simulink model "UAM_Flight_control"  (R2024b)
settings: Solver=FixedStepAuto  StartTime=0.0  StopTime=inf  RelTol=1e-3  EnableMultiTasking=on
undefined symbols (not defined in the file): CityMission, control, controlParams, ControlSampleTime, Cruise_a, DiscIntNeverNeededParam, Earth, FixedWingMission, flightState, FSState, FWControlParams, FWTrimSpeed, HoverMission, params, position, R_WAYPOINTTRANSITION, TransitionMission, uavParam, Vt, w_trim, WGS84, zGround
libraries: slpidlib x56, simulink x32, uavalgslib x7, robotcorelib x2, simulink_extras x2, mspfiltlib x1, aerolibtransform2 x1
(part 5 of 13)

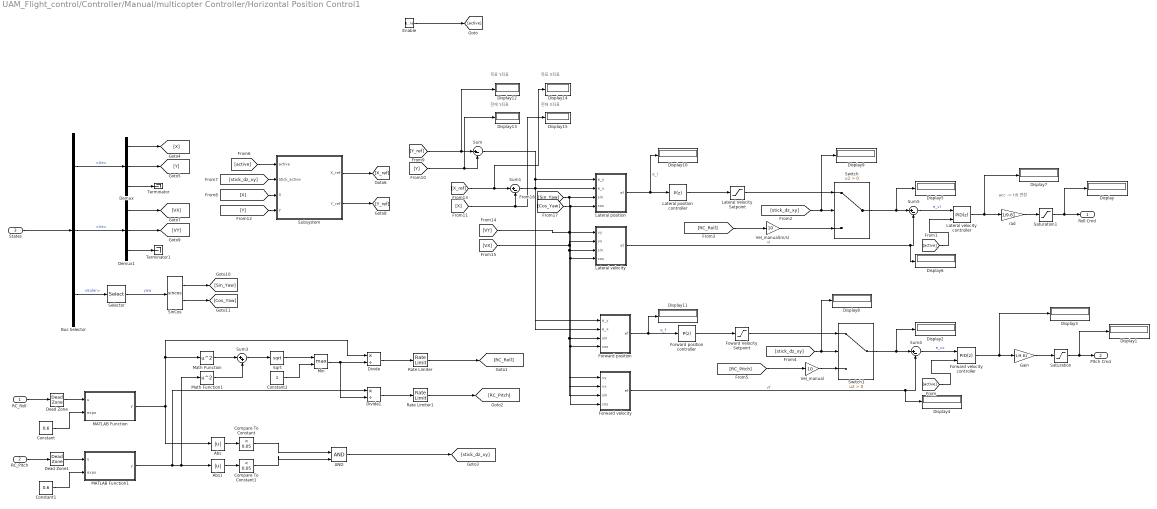
== system UAM_Flight_control/Controller/Manual/multicopter Controller/Horizontal Position Control1 ==
  note: 현재 X좌표
  note: 현재 Y좌표
  note: acc -> tilt 변환
  note: 목표 X좌표
  note: 목표 Y좌표
  RC_Roll : Inport
  RC_Pitch : Inport  Port=2
  States : Inport  Port=3
  Enable : EnablePort  StatesWhenEnabling=reset  ShowOutputPort=on
  AND : Logic  IconShape=distinctive  AllPortsSameDT=off  OutDataTypeStr=boolean
  Abs : Abs  SaturateOnIntegerOverflow=off
  Abs1 : Abs  SaturateOnIntegerOverflow=off
  Bus Selector : BusSelector  OutputSignals=Xe,Ve,Euler
  Compare To Constant : simulink/Logic and Bit Operations/Compare To Constant  relop=<  const=0.05  OutDataTypeStr=boolean
  Compare To Constant1 : simulink/Logic and Bit Operations/Compare To Constant  relop=<  const=0.05  OutDataTypeStr=boolean
  Constant : Constant  Value=0.6
  Constant1 : Constant  Value=0.6
  Constant2 : Constant
  Dead Zone : DeadZone  LowerValue=-0.1  UpperValue=0.1
  Dead Zone1 : DeadZone  LowerValue=-0.1  UpperValue=0.1
  Demux : Demux  Outputs=3
  Demux1 : Demux  Outputs=3
  Display{,1..15} (16 alike) : Display
  Divide : Product  Inputs=*/
  Divide1 : Product  Inputs=*/
  Forward position : Subsystem
  Forward position controller : slpidlib/PID Controller  Controller=P  Form=Parallel  TimeDomain=Discrete-time  UseExternalTs=off  SampleTime=-1  IntegratorMethod=Forward Euler  FilterMethod=Forward Euler  ControllerParametersSource=internal  P=controlParams.P_X  I=controlParams.I_X  UseKiTs=off  D=controlParams.D_X  UseExternalDerivativeSource=off  N=controlParams.N_X  UseFilter=on  TunerSelectOption=Transfer Function Based (PID Tuner App)  InitialConditionSource=internal  InitialConditionForIntegrator=0  InitialConditionForFilter=0  DifferentiatorICPrevScaledInput=0  ExternalReset=none  TrackingMode=off  Kt=1  LimitOutput=off  SatLimitsSource=internal  UpperSaturationLimit=inf  LowerSaturationLimit=-inf  LinearizeAsGain=on  AntiWindupMode=none  Kb=1  LimitIntegrator=off  UpperIntegratorSaturationLimit=inf  LowerIntegratorSaturationLimit=-inf  POutMin=[]  POutMax=[]  IOutMin=[]  IOutMax=[]  DOutMin=[]  DOutMax=[]  NOutMin=[]  NOutMax=[]  SumOutMin=[]  SumOutMax=[]  SaturationOutMin=[]  SaturationOutMax=[]  PParamMin=[]  PParamMax=[]  IParamMin=[]  IParamMax=[]  DParamMin=[]  DParamMax=[]  NParamMin=[]  NParamMax=[]  KbParamMin=[]  KbParamMax=[]  KtParamMin=[]  KtParamMax=[]  KbOutMin=[]  KbOutMax=[]  KtOutMin=[]  KtOutMax=[]  IntegratorOutMin=[]  IntegratorOutMax=[]  FilterOutMin=[]  FilterOutMax=[]  SumI1OutMin=[]  SumI1OutMax=[]  SumI2OutMin=[]  SumI2OutMax=[]  SumI3OutMin=[]  SumI3OutMax=[]  SumI4OutMin=[]  SumI4OutMax=[]  SumDOutMin=[]  SumDOutMax=[]  DifferentiatorOutMin=[]  DifferentiatorOutMax=[]  FilterDiffOutCoefMin=[]  FilterDiffOutCoefMax=[]  ReciprocalOutMin=[]  ReciprocalOutMax=[]  SumDenOutMin=[]  SumDenOutMax=[]  SumNumOutMin=[]  SumNumOutMax=[]  DivideOutMin=[]  DivideOutMax=[]  UdiffTsProdOutMin=[]  UdiffTsProdOutMax=[]  NTsProdOutMin=[]  NTsProdOutMax=[]  UintegralTsProdOutMin=[]  UintegralTsProdOutMax=[]  UngainTsProdOutMin=[]  UngainTsProdOutMax=[]  ClampingZeroOutDataTypeStr=Inherit: Inherit via back propagation  ClampingZeroOutMin=[]  ClampingZeroOutMax=[]  FilterDenConstantOutDataTypeStr=Inherit: Inherit via back propagation  FilterDenConstantOutMin=[]  FilterDenConstantOutMax=[]  PCopyOutDataTypeStr=Inherit: Inherit via back propagation  PCopyOutMin=[]  PCopyOutMax=[]  NCopyOutDataTypeStr=Inherit: Inherit via back propagation  NCopyOutMin=[]  NCopyOutMax=[]  IntegratorContinuousStateAttributes=''  IntegratorStateMustResolveToSignalObject=off  IntegratorRTWStateStorageClass=Auto  FilterContinuousStateAttributes=''  FilterStateMustResolveToSignalObject=off  FilterRTWStateStorageClass=Auto  ParallelPVariant=InternalParameters  IdealPVariant=Disabled  IVariant=Disabled  DVariant=Disabled  IntegratorVariant=Disabled  SatVariant=Disabled  AWVariant=Disabled  PCopyVariant=Disabled  TRVariant=Disabled  FdbkBlocksVariant=Forward  IdealPFdbkVariant=Disabled  SatFdbkVariant=Disabled  DerivativeFilterVariant=Disabled  NVariant=Disabled  NCopyVariant=Disabled_SignalSpec  FilterICVariant=Disabled  IntegratorICVariant=Disabled  ExternalResetVariant=Disabled  TRSumVariant=Passthrough  SumFdbkVariant=Disabled  SumVariant=Passthrough_P  TsampFilterVariant=InternalTs  TsampNgainVariant=Passthrough  TsampIntegralVariant=Disabled_SignalSpec  ExternalSaturationOutDataTypeStr=Inherit: Same as second input  DerivativeSourceVariant=Disabled  PreIntVariant=InternalPreInt
  Forward velocity : Subsystem
  Forward velocity controller : slpidlib/PID Controller  Controller=PID  Form=Parallel  TimeDomain=Discrete-time  UseExternalTs=off  SampleTime=-1  IntegratorMethod=Forward Euler  FilterMethod=Forward Euler  ControllerParametersSource=internal  P=controlParams.P_VX  I=controlParams.I_VX  UseKiTs=off  D=controlParams.D_VX  UseExternalDerivativeSource=off  N=controlParams.N_VX  UseFilter=on  TunerSelectOption=Transfer Function Based (PID Tuner App)  InitialConditionSource=internal  InitialConditionForIntegrator=0  InitialConditionForFilter=0  DifferentiatorICPrevScaledInput=0  ExternalReset=rising  TrackingMode=off  Kt=1  LimitOutput=on  SatLimitsSource=internal  UpperSaturationLimit=5  LowerSaturationLimit=-5  LinearizeAsGain=on  AntiWindupMode=clamping  Kb=1  LimitIntegrator=on  UpperIntegratorSaturationLimit=2  LowerIntegratorSaturationLimit=-2  POutMin=[]  POutMax=[]  IOutMin=[]  IOutMax=[]  DOutMin=[]  DOutMax=[]  NOutMin=[]  NOutMax=[]  SumOutMin=[]  SumOutMax=[]  SaturationOutMin=[]  SaturationOutMax=[]  PParamMin=[]  PParamMax=[]  IParamMin=[]  IParamMax=[]  DParamMin=[]  DParamMax=[]  NParamMin=[]  NParamMax=[]  KbParamMin=[]  KbParamMax=[]  KtParamMin=[]  KtParamMax=[]  KbOutMin=[]  KbOutMax=[]  KtOutMin=[]  KtOutMax=[]  IntegratorOutMin=[]  IntegratorOutMax=[]  FilterOutMin=[]  FilterOutMax=[]  SumI1OutMin=[]  SumI1OutMax=[]  SumI2OutMin=[]  SumI2OutMax=[]  SumI3OutMin=[]  SumI3OutMax=[]  SumI4OutMin=[]  SumI4OutMax=[]  SumDOutMin=[]  SumDOutMax=[]  DifferentiatorOutMin=[]  DifferentiatorOutMax=[]  FilterDiffOutCoefMin=[]  FilterDiffOutCoefMax=[]  ReciprocalOutMin=[]  ReciprocalOutMax=[]  SumDenOutMin=[]  SumDenOutMax=[]  SumNumOutMin=[]  SumNumOutMax=[]  DivideOutMin=[]  DivideOutMax=[]  UdiffTsProdOutMin=[]  UdiffTsProdOutMax=[]  NTsProdOutMin=[]  NTsProdOutMax=[]  UintegralTsProdOutMin=[]  UintegralTsProdOutMax=[]  UngainTsProdOutMin=[]  UngainTsProdOutMax=[]  ClampingZeroOutDataTypeStr=Inherit: Inherit via back propagation  ClampingZeroOutMin=[]  ClampingZeroOutMax=[]  FilterDenConstantOutDataTypeStr=Inherit: Inherit via back propagation  FilterDenConstantOutMin=[]  FilterDenConstantOutMax=[]  PCopyOutDataTypeStr=Inherit: Inherit via back propagation  PCopyOutMin=[]  PCopyOutMax=[]  NCopyOutDataTypeStr=Inherit: Inherit via back propagation  NCopyOutMin=[]  NCopyOutMax=[]  IntegratorContinuousStateAttributes=''  IntegratorStateMustResolveToSignalObject=off  IntegratorRTWStateStorageClass=Auto  FilterContinuousStateAttributes=''  FilterStateMustResolveToSignalObject=off  FilterRTWStateStorageClass=Auto  ParallelPVariant=InternalParameters  IdealPVariant=Disabled  IVariant=InternalParameters  DVariant=InternalParameters  IntegratorVariant=Discrete  SatVariant=Enabled  AWVariant=DiscClampingParallel  PCopyVariant=Disabled  TRVariant=Disabled  FdbkBlocksVariant=Forward  IdealPFdbkVariant=Disabled  SatFdbkVariant=Disabled  DerivativeFilterVariant=ForwardEulerFilter  NVariant=InternalParameters  NCopyVariant=Disabled  FilterICVariant=InternalICsFilter  IntegratorICVariant=InternalICs  ExternalResetVariant=ExternalReset  TRSumVariant=Passthrough  SumFdbkVariant=Disabled  SumVariant=Sum_PID  TsampFilterVariant=InternalTs  TsampNgainVariant=Passthrough  TsampIntegralVariant=Disabled_SignalSpec  ExternalSaturationOutDataTypeStr=Inherit: Same as second input  DerivativeSourceVariant=ErrorSignal  PreIntVariant=InternalPreInt
  Foward Velocity Setpoint : Saturate  UpperLimit=10  LowerLimit=-10
  Gain : Gain  Gain=1/9.81
  Lateral Velocity Setpoint : Saturate  UpperLimit=10  LowerLimit=-10
  Lateral position : Subsystem
  Lateral position controller : slpidlib/PID Controller  Controller=P  Form=Parallel  TimeDomain=Discrete-time  UseExternalTs=off  SampleTime=-1  IntegratorMethod=Forward Euler  FilterMethod=Forward Euler  ControllerParametersSource=internal  P=controlParams.P_Y  I=controlParams.I_Y  UseKiTs=off  D=controlParams.D_Y  UseExternalDerivativeSource=off  N=controlParams.N_Y  UseFilter=on  TunerSelectOption=Transfer Function Based (PID Tuner App)  InitialConditionSource=internal  InitialConditionForIntegrator=0  InitialConditionForFilter=0  DifferentiatorICPrevScaledInput=0  ExternalReset=none  TrackingMode=off  Kt=1  LimitOutput=on  SatLimitsSource=internal  UpperSaturationLimit=5  LowerSaturationLimit=-5  LinearizeAsGain=on  AntiWindupMode=clamping  Kb=1  LimitIntegrator=off  UpperIntegratorSaturationLimit=inf  LowerIntegratorSaturationLimit=-inf  POutMin=[]  POutMax=[]  IOutMin=[]  IOutMax=[]  DOutMin=[]  DOutMax=[]  NOutMin=[]  NOutMax=[]  SumOutMin=[]  SumOutMax=[]  SaturationOutMin=[]  SaturationOutMax=[]  PParamMin=[]  PParamMax=[]  IParamMin=[]  IParamMax=[]  DParamMin=[]  DParamMax=[]  NParamMin=[]  NParamMax=[]  KbParamMin=[]  KbParamMax=[]  KtParamMin=[]  KtParamMax=[]  KbOutMin=[]  KbOutMax=[]  KtOutMin=[]  KtOutMax=[]  IntegratorOutMin=[]  IntegratorOutMax=[]  FilterOutMin=[]  FilterOutMax=[]  SumI1OutMin=[]  SumI1OutMax=[]  SumI2OutMin=[]  SumI2OutMax=[]  SumI3OutMin=[]  SumI3OutMax=[]  SumI4OutMin=[]  SumI4OutMax=[]  SumDOutMin=[]  SumDOutMax=[]  DifferentiatorOutMin=[]  DifferentiatorOutMax=[]  FilterDiffOutCoefMin=[]  FilterDiffOutCoefMax=[]  ReciprocalOutMin=[]  ReciprocalOutMax=[]  SumDenOutMin=[]  SumDenOutMax=[]  SumNumOutMin=[]  SumNumOutMax=[]  DivideOutMin=[]  DivideOutMax=[]  UdiffTsProdOutMin=[]  UdiffTsProdOutMax=[]  NTsProdOutMin=[]  NTsProdOutMax=[]  UintegralTsProdOutMin=[]  UintegralTsProdOutMax=[]  UngainTsProdOutMin=[]  UngainTsProdOutMax=[]  ClampingZeroOutDataTypeStr=Inherit: Inherit via back propagation  ClampingZeroOutMin=[]  ClampingZeroOutMax=[]  FilterDenConstantOutDataTypeStr=Inherit: Inherit via back propagation  FilterDenConstantOutMin=[]  FilterDenConstantOutMax=[]  PCopyOutDataTypeStr=Inherit: Inherit via back propagation  PCopyOutMin=[]  PCopyOutMax=[]  NCopyOutDataTypeStr=Inherit: Inherit via back propagation  NCopyOutMin=[]  NCopyOutMax=[]  IntegratorContinuousStateAttributes=''  IntegratorStateMustResolveToSignalObject=off  IntegratorRTWStateStorageClass=Auto  FilterContinuousStateAttributes=''  FilterStateMustResolveToSignalObject=off  FilterRTWStateStorageClass=Auto  ParallelPVariant=InternalParameters  IdealPVariant=Disabled  IVariant=Disabled  DVariant=Disabled  IntegratorVariant=Disabled  SatVariant=Enabled  AWVariant=Disabled  PCopyVariant=Disabled  TRVariant=Disabled  FdbkBlocksVariant=Forward  IdealPFdbkVariant=Disabled  SatFdbkVariant=Disabled  DerivativeFilterVariant=Disabled  NVariant=Disabled  NCopyVariant=Disabled_SignalSpec  FilterICVariant=Disabled  IntegratorICVariant=Disabled  ExternalResetVariant=Disabled  TRSumVariant=Passthrough  SumFdbkVariant=Disabled  SumVariant=Passthrough_P  TsampFilterVariant=InternalTs  TsampNgainVariant=Passthrough  TsampIntegralVariant=Disabled_SignalSpec  ExternalSaturationOutDataTypeStr=Inherit: Same as second input  DerivativeSourceVariant=Disabled  PreIntVariant=InternalPreInt
  Lateral velocity : Subsystem
  Lateral velocity controller : slpidlib/PID Controller  Controller=PID  Form=Parallel  TimeDomain=Discrete-time  UseExternalTs=off  SampleTime=-1  IntegratorMethod=Forward Euler  FilterMethod=Forward Euler  ControllerParametersSource=internal  P=controlParams.P_VY  I=controlParams.I_VY  UseKiTs=off  D=controlParams.D_VY  UseExternalDerivativeSource=off  N=controlParams.N_VY  UseFilter=on  TunerSelectOption=Transfer Function Based (PID Tuner App)  InitialConditionSource=internal  InitialConditionForIntegrator=0  InitialConditionForFilter=0  DifferentiatorICPrevScaledInput=0  ExternalReset=rising  TrackingMode=off  Kt=1  LimitOutput=on  SatLimitsSource=internal  UpperSaturationLimit=5  LowerSaturationLimit=-5  LinearizeAsGain=on  AntiWindupMode=clamping  Kb=1  LimitIntegrator=on  UpperIntegratorSaturationLimit=2  LowerIntegratorSaturationLimit=-2  POutMin=[]  POutMax=[]  IOutMin=[]  IOutMax=[]  DOutMin=[]  DOutMax=[]  NOutMin=[]  NOutMax=[]  SumOutMin=[]  SumOutMax=[]  SaturationOutMin=[]  SaturationOutMax=[]  PParamMin=[]  PParamMax=[]  IParamMin=[]  IParamMax=[]  DParamMin=[]  DParamMax=[]  NParamMin=[]  NParamMax=[]  KbParamMin=[]  KbParamMax=[]  KtParamMin=[]  KtParamMax=[]  KbOutMin=[]  KbOutMax=[]  KtOutMin=[]  KtOutMax=[]  IntegratorOutMin=[]  IntegratorOutMax=[]  FilterOutMin=[]  FilterOutMax=[]  SumI1OutMin=[]  SumI1OutMax=[]  SumI2OutMin=[]  SumI2OutMax=[]  SumI3OutMin=[]  SumI3OutMax=[]  SumI4OutMin=[]  SumI4OutMax=[]  SumDOutMin=[]  SumDOutMax=[]  DifferentiatorOutMin=[]  DifferentiatorOutMax=[]  FilterDiffOutCoefMin=[]  FilterDiffOutCoefMax=[]  ReciprocalOutMin=[]  ReciprocalOutMax=[]  SumDenOutMin=[]  SumDenOutMax=[]  SumNumOutMin=[]  SumNumOutMax=[]  DivideOutMin=[]  DivideOutMax=[]  UdiffTsProdOutMin=[]  UdiffTsProdOutMax=[]  NTsProdOutMin=[]  NTsProdOutMax=[]  UintegralTsProdOutMin=[]  UintegralTsProdOutMax=[]  UngainTsProdOutMin=[]  UngainTsProdOutMax=[]  ClampingZeroOutDataTypeStr=Inherit: Inherit via back propagation  ClampingZeroOutMin=[]  ClampingZeroOutMax=[]  FilterDenConstantOutDataTypeStr=Inherit: Inherit via back propagation  FilterDenConstantOutMin=[]  FilterDenConstantOutMax=[]  PCopyOutDataTypeStr=Inherit: Inherit via back propagation  PCopyOutMin=[]  PCopyOutMax=[]  NCopyOutDataTypeStr=Inherit: Inherit via back propagation  NCopyOutMin=[]  NCopyOutMax=[]  IntegratorContinuousStateAttributes=''  IntegratorStateMustResolveToSignalObject=off  IntegratorRTWStateStorageClass=Auto  FilterContinuousStateAttributes=''  FilterStateMustResolveToSignalObject=off  FilterRTWStateStorageClass=Auto  ParallelPVariant=InternalParameters  IdealPVariant=Disabled  IVariant=InternalParameters  DVariant=InternalParameters  IntegratorVariant=Discrete  SatVariant=Enabled  AWVariant=DiscClampingParallel  PCopyVariant=Disabled  TRVariant=Disabled  FdbkBlocksVariant=Forward  IdealPFdbkVariant=Disabled  SatFdbkVariant=Disabled  DerivativeFilterVariant=ForwardEulerFilter  NVariant=InternalParameters  NCopyVariant=Disabled  FilterICVariant=InternalICsFilter  IntegratorICVariant=InternalICs  ExternalResetVariant=ExternalReset  TRSumVariant=Passthrough  SumFdbkVariant=Disabled  SumVariant=Sum_PID  TsampFilterVariant=InternalTs  TsampNgainVariant=Passthrough  TsampIntegralVariant=Disabled_SignalSpec  ExternalSaturationOutDataTypeStr=Inherit: Same as second input  DerivativeSourceVariant=ErrorSignal  PreIntVariant=InternalPreInt
  MATLAB Function : MATLAB Function  TreatAsAtomicUnit=on
  MATLAB Function1 : MATLAB Function  TreatAsAtomicUnit=on
  Math Function : Math  Operator=square
  Math Function1 : Math  Operator=square
  Min : MinMax  Function=max  Inputs=2
  Rate Limiter : RateLimiter  SampleTimeMode=inherited
  Rate Limiter1 : RateLimiter  SampleTimeMode=inherited
  Saturation : Saturate  UpperLimit=0.51  LowerLimit=-0.51
  Saturation1 : Saturate  UpperLimit=0.51  LowerLimit=-0.51
  Selector : Selector  InputPortWidth=3  IndexOptions=Index vector (dialog)  Indices=[3]  OutputSizes=1
  SinCos : Trigonometry  Operator=sincos
  Sqrt : Sqrt
  Subsystem : Subsystem
  Sum{,1,4..5} (4 alike) : Sum  Inputs=|+-
  Sum3 : Sum  Inputs=|++
  Switch : Switch  Criteria=u2 > Threshold  SaturateOnIntegerOverflow=off  InputSameDT=off
  Switch1 : Switch  Criteria=u2 > Threshold  SaturateOnIntegerOverflow=off  InputSameDT=off
  Terminator : Terminator
  Terminator1 : Terminator
  Vel_manual : Gain  Gain=10
  Vel_manual(m/s) : Gain  Gain=10
  rad : Gain  Gain=1/9.81
  Roll Cmd : Outport
  Pitch Cmd : Outport  Port=2
  wires:
  Saturation1/1 -> Roll Cmd/1, Display/1
  Saturation/1 -> Pitch Cmd/1, Display1/1
  Forward velocity controller/1 -> Display3/1, Gain/1
  States/1 -> Bus Selector/1
  Bus Selector/3 -> Selector/1  "<Euler>"
  Selector/1 -> SinCos/1  "yaw"
  Demux/3 -> Terminator/1
  Demux1/3 -> Terminator1/1
  Lateral velocity/1(el) -> Display6/1, Sum5/2  "vl"
  Sum4/1 -> Forward velocity controller/1  "e_vx"
  Bus Selector/1 -> Demux/1  "<Xe>"
  Bus Selector/2 -> Demux1/1  "<Ve>"
  Enable/1 -> [active]
  [active] -> Forward velocity controller/2
  [active] -> Lateral velocity controller/2
  rad/1 -> Saturation1/1
  Gain/1 -> Saturation/1
  RC_Roll/1 -> Dead Zone/1
  RC_Pitch/1 -> Dead Zone1/1
  Abs/1 -> Compare To Constant/1
  Compare To Constant/1 -> AND/1
  Abs1/1 -> Compare To Constant1/1
  Compare To Constant1/1 -> AND/2
  [stick_dz_xy] -> Display9/1, Switch/2
  Vel_manual(m/s)/1 -> Switch/3
  [RC_Roll] -> Vel_manual(m/s)/1
  Lateral Velocity Setpoint/1 -> Switch/1
  Switch/1 -> Display5/1, Sum5/1
  Sum5/1 -> Lateral velocity controller/1  "e_vl"
  Lateral velocity controller/1 -> Display7/1, rad/1
  [stick_dz_xy] -> Display8/1, Switch1/2
  Foward Velocity Setpoint/1 -> Switch1/1
  Vel_manual/1 -> Switch1/3
  [RC_Pitch] -> Vel_manual/1
  Switch1/1 -> Display2/1, Sum4/1
  Forward velocity/1(ef) -> Display4/1, Sum4/2  "vf"
  Demux/1 -> [X]
  Demux/2 -> [Y]
  [active] -> Subsystem/1(active)
  [stick_dz_xy] -> Subsystem/2(Stick_active)
  Subsystem/1(X_ref) -> [X_ref]
  [Y] -> Subsystem/4(Y)
  [X] -> Subsystem/3(X)
  Subsystem/2(Y_ref) -> [Y_ref]
  Demux1/1 -> [VX]
  Demux1/2 -> [VY]
  SinCos/1 -> [Sin_Yaw]
  SinCos/2 -> [Cos_Yaw]
  Sum/1 -> Forward position/1(e_y), Lateral position/1(e_y)
  Sum1/1 -> Forward position/2(e_x), Lateral position/2(e_x)
  [Sin_Yaw] -> Lateral position/3(sin), Lateral velocity/3(sin), Forward velocity/3(sin), Forward position/3(sin)
  [Cos_Yaw] -> Lateral position/4(cos), Lateral velocity/4(cos), Forward position/4(cos), Forward velocity/4(cos)
  Forward position/1(ef) -> Display11/1, Forward position controller/1  "e_f"
  Lateral position/1(el) -> Display10/1, Lateral position controller/1  "e_l"
  Dead Zone/1 -> MATLAB Function/1(u)
  MATLAB Function/1(y) -> Divide/1, Math Function/1, Abs/1
  MATLAB Function1/1(y) -> Divide1/1, Math Function1/1, Abs1/1
  Dead Zone1/1 -> MATLAB Function1/1(u)
  Constant/1 -> MATLAB Function/2(expo)
  Constant1/1 -> MATLAB Function1/2(expo)
  Math Function/1 -> Sum3/1
  Math Function1/1 -> Sum3/2
  Sum3/1 -> Sqrt/1
  Sqrt/1 -> Min/1
  Constant2/1 -> Min/2
  Min/1 -> Divide1/2, Divide/2
  Divide1/1 -> Rate Limiter1/1
  Divide/1 -> Rate Limiter/1
  Rate Limiter/1 -> [RC_Roll]
  Rate Limiter1/1 -> [RC_Pitch]
  AND/1 -> [stick_dz_xy]
  Lateral position controller/1 -> Lateral Velocity Setpoint/1
  Forward position controller/1 -> Foward Velocity Setpoint/1
  [Y_ref] -> Display12/1, Sum/1
  [Y] -> Display13/1, Sum/2
  [X_ref] -> Display14/1, Sum1/1
  [X] -> Display15/1, Sum1/2
  [VY] -> Forward velocity/1(vy), Lateral velocity/1(vy)
  [VX] -> Lateral velocity/2(vx), Forward velocity/2(vx)

== system UAM_Flight_control/Controller/Manual/multicopter Controller/Organize Inputs ==
  forward command : Inport
  commanded phi torque : Inport  Port=2
  commanded theta torque : Inport  Port=3
  commanded psi torque : Inport  Port=4
  commanded thrust : Inport  Port=5
  Out Bus Element : Outport  PortName=MixerCommands  Element=w_phi
  Out Bus Element1 : Outport  PortName=MixerCommands  Element=w_theta
  Out Bus Element2 : Outport  PortName=MixerCommands  Element=w_psi
  Out Bus Element3 : Outport  PortName=MixerCommands  Element=w_z
  Out Bus Element4 : Outport  PortName=MixerCommands  Element=l_x
  wires:
  commanded theta torque/1 -> Out Bus Element1/1  "theta"
  commanded psi torque/1 -> Out Bus Element2/1  "psi"
  commanded thrust/1 -> Out Bus Element3/1  "thrust"
  forward command/1 -> Out Bus Element4/1  "foward"
  commanded phi torque/1 -> Out Bus Element/1  "phi"

== system UAM_Flight_control/Controller/Manual/multicopter Controller/RC_Normalization ==
  note: -1 ~ 1 정규화
  note: 0 ~ 1 정규화
  RC : Inport
  Bias : Bias  Bias=-1500  SaturateOnIntegerOverflow=off
  Bias1 : Bias  Bias=-1000  SaturateOnIntegerOverflow=off
  Demux : Demux  Outputs=10
  Demux2 : Demux  Outputs=3
  Gain : Gain  Gain=1/500
  Gain1 : Gain  Gain=1/1000
  Mux1 : Mux  Inputs=3
  Saturation : Saturate  UpperLimit=1  LowerLimit=0
  Terminator{1..6} (6 alike) : Terminator
  Rollcmd : Outport
  Pitchcmd : Outport  Port=2
  Yawcmd : Outport  Port=3
  Throttlecmd : Outport  Port=4
  wires:
  Demux/7 -> Terminator3/1
  Bias1/1 -> Gain1/1
  Demux/5 -> Terminator1/1
  Demux/4 -> Mux1/3
  Bias/1 -> Gain/1
  Demux/1 -> Mux1/1
  RC/1 -> Demux/1
  Gain1/1 -> Saturation/1
  Demux/3 -> Bias1/1
  Demux/9 -> Terminator5/1
  Saturation/1 -> Throttlecmd/1
  Demux/6 -> Terminator2/1
  Gain/1 -> Demux2/1
  Demux/8 -> Terminator4/1
  Demux/10 -> Terminator6/1
  Demux2/2 -> Pitchcmd/1
  Demux2/1 -> Rollcmd/1
  Mux1/1 -> Bias/1
  Demux/2 -> Mux1/2
  Demux2/3 -> Yawcmd/1

== system UAM_Flight_control/Controller/Manual/multicopter Controller/Subsystem ==
  In1 : Inport
  Enable : EnablePort
  Display10 : Display
  Out1 : Outport
  wires:
  In1/1 -> Display10/1, Out1/1

== system UAM_Flight_control/Flightmode/Auto/Guidance Mode Selector/GuidanceLogic.WP/Back Transition Guard ==
  note: Set previous waypoint to current location if the UAV has just exited back transition
  Poses : Inport
  FromWP : Inport  Port=2
  Bus Selector : BusSelector  OutputSignals=mode
  Bus Selector1 : BusSelector  OutputSignals=position,params,mode
  Constant : Constant  Value=6
  Equal : RelationalOperator  Operator===  OutDataTypeStr=boolean  RndMeth=Simplest  InputSameDT=off
  Switch : Switch  Criteria=u2 > Threshold  SaturateOnIntegerOverflow=off  InputSameDT=off
  Triggered Subsystem : Subsystem  TreatAsAtomicUnit=on
  Out Bus Element2 : Outport  PortName=PrevWP  Element=mode
  Out Bus Element : Outport  PortName=PrevWP  Element=position
  Out Bus Element1 : Outport  PortName=PrevWP  Element=params
  wires:
  FromWP/1 -> Bus Selector1/1, Bus Selector/1
  Bus Selector/1 -> Equal/2  "<mode>"
  Constant/1 -> Equal/1
  Equal/1 -> Switch/2, Triggered Subsystem/Trigger
  Poses/1 -> Triggered Subsystem/1(Poses)
  Triggered Subsystem/1(HoldPositionValue) -> Switch/1
  Switch/1 -> Out Bus Element/1
  Bus Selector1/2 -> Out Bus Element1/1  "<params>"
  Bus Selector1/3 -> Out Bus Element2/1  "<mode>"
  Bus Selector1/1 -> Switch/3  "<position>"

== system UAM_Flight_control/Flightmode/Auto/Guidance Mode Selector/GuidanceLogic.WP/Dist2WP ==
  Pose : Inport
  FromWP : Inport  Port=2
  ToWP : Inport  Port=3
  Bus Selector : BusSelector  OutputSignals=position
  Bus Selector1 : BusSelector  OutputSignals=position
  Demux : Demux  Outputs=[3 1]
  Dot Product : DotProduct  OutDataTypeStr=Inherit: Inherit via internal rule
  Subsystem : Subsystem
  Sum : Sum  Inputs=|-+
  Sum1 : Sum  Inputs=|+-
  Terminator : Terminator
  Dist : Outport
  wires:
  Sum1/1 -> Subsystem/1(V)
  Demux/2 -> Terminator/1
  Bus Selector/1 -> Sum/2, Sum1/1  "<position>"
  Demux/1 -> Sum/1
  Bus Selector1/1 -> Sum1/2  "<position>"
  Sum/1 -> Dot Product/1
  Subsystem/1(V_unit) -> Dot Product/2
  Pose/1 -> Demux/1
  Dot Product/1 -> Dist/1
  ToWP/1 -> Bus Selector/1
  FromWP/1 -> Bus Selector1/1

== system UAM_Flight_control/GNC/Navigation/LLA2Local/Enabled Subsystem ==
  LLA : Inport
  homeLLA : Inport  Port=2
  Enable : EnablePort
  Constant1 : Constant  Value=0
  Demux1 : Demux  Outputs=[2 1]
  Demux2 : Demux  Outputs=[2 1]
  Display : Display
  Display1 : Display
  Display2 : Display
  LLA to Flat Earth1 : aerolibtransform2/LLA to Flat Earth  units=Metric (MKS)  ptype=Earth (WGS84)  F=1/298.257223563  R=6378137  refPosPort=on  LL0=[0,0]  psi=0
  Reshape : Reshape  OutputDimensionality=Customize  OutputDimensions=[2 1]
  Reshape1 : Reshape  OutputDimensionality=Customize  OutputDimensions=[2 1]
  Xe : Outport
  wires:
  Constant1/1 -> LLA to Flat Earth1/5
  LLA to Flat Earth1/1 -> Display2/1, Xe/1  "Xe"
  Demux1/2 -> LLA to Flat Earth1/2
  Demux1/1 -> Reshape/1
  homeLLA/1 -> Display/1, Demux2/1
  LLA/1 -> Display1/1, Demux1/1
  Demux2/2 -> LLA to Flat Earth1/3
  Demux2/1 -> Reshape1/1
  Reshape/1 -> LLA to Flat Earth1/1
  Reshape1/1 -> LLA to Flat Earth1/4

== system UAM_Flight_control/Controller/Auto1/Fixed Wing Controller/Subsystem/AER from Path Manager ==
  In1 : Inport
  Enable : EnablePort
  Out1 : Outport
  wires:
  In1/1 -> Out1/1

== system UAM_Flight_control/Controller/Auto1/Fixed Wing Controller/Subsystem/Airspeed-Altitude Controller ==
  note: Airspeed and altitude are controlled independently
      | by ignoring their coupled dynamics.
  Airspeed SP : Inport
  Altitude SP : Inport  Port=2
  Climb Rate SP : Inport  Port=3
  Airspeed : Inport  Port=4
  xyz : Inport  Port=5
  vxyz : Inport  Port=6
  Control Mode : EnablePort  ShowOutputPort=on
  Airspeed Controller : slpidlib/PID Controller  Controller=PID  Form=Parallel  TimeDomain=Discrete-time  UseExternalTs=off  SampleTime=ControlSampleTime  IntegratorMethod=Trapezoidal  FilterMethod=Forward Euler  ControllerParametersSource=internal  P=FWControlParams.P_AIRSPD  I=FWControlParams.I_AIRSPD  UseKiTs=off  D=FWControlParams.D_AIRSPD  UseExternalDerivativeSource=off  N=FWControlParams.N_AIRSPD  UseFilter=on  TunerSelectOption=Transfer Function Based (PID Tuner App)  InitialConditionSource=internal  InitialConditionForIntegrator=0  InitialConditionForFilter=0  DifferentiatorICPrevScaledInput=0  ExternalReset=none  TrackingMode=off  Kt=1  LimitOutput=off  SatLimitsSource=internal  UpperSaturationLimit=Inf  LowerSaturationLimit=0  LinearizeAsGain=on  AntiWindupMode=clamping  Kb=1  LimitIntegrator=off  UpperIntegratorSaturationLimit=inf  LowerIntegratorSaturationLimit=-inf  POutMin=[]  POutMax=[]  IOutMin=[]  IOutMax=[]  DOutMin=[]  DOutMax=[]  NOutMin=[]  NOutMax=[]  SumOutMin=[]  SumOutMax=[]  SaturationOutMin=[]  SaturationOutMax=[]  PParamMin=[]  PParamMax=[]  IParamMin=[]  IParamMax=[]  DParamMin=[]  DParamMax=[]  NParamMin=[]  NParamMax=[]  KbParamMin=[]  KbParamMax=[]  KtParamMin=[]  KtParamMax=[]  KbOutMin=[]  KbOutMax=[]  KtOutMin=[]  KtOutMax=[]  IntegratorOutMin=[]  IntegratorOutMax=[]  FilterOutMin=[]  FilterOutMax=[]  SumI1OutMin=[]  SumI1OutMax=[]  SumI2OutMin=[]  SumI2OutMax=[]  SumI3OutMin=[]  SumI3OutMax=[]  SumI4OutMin=[]  SumI4OutMax=[]  SumDOutMin=[]  SumDOutMax=[]  DifferentiatorOutMin=[]  DifferentiatorOutMax=[]  FilterDiffOutCoefMin=[]  FilterDiffOutCoefMax=[]  ReciprocalOutMin=[]  ReciprocalOutMax=[]  SumDenOutMin=[]  SumDenOutMax=[]  SumNumOutMin=[]  SumNumOutMax=[]  DivideOutMin=[]  DivideOutMax=[]  UdiffTsProdOutMin=[]  UdiffTsProdOutMax=[]  NTsProdOutMin=[]  NTsProdOutMax=[]  UintegralTsProdOutMin=[]  UintegralTsProdOutMax=[]  UngainTsProdOutMin=[]  UngainTsProdOutMax=[]  ClampingZeroOutDataTypeStr=Inherit: Inherit via back propagation  ClampingZeroOutMin=[]  ClampingZeroOutMax=[]  FilterDenConstantOutDataTypeStr=Inherit: Inherit via back propagation  FilterDenConstantOutMin=[]  FilterDenConstantOutMax=[]  PCopyOutDataTypeStr=Inherit: Inherit via back propagation  PCopyOutMin=[]  PCopyOutMax=[]  NCopyOutDataTypeStr=Inherit: Inherit via back propagation  NCopyOutMin=[]  NCopyOutMax=[]  IntegratorContinuousStateAttributes=''  IntegratorStateMustResolveToSignalObject=off  IntegratorRTWStateStorageClass=Auto  FilterContinuousStateAttributes=''  FilterStateMustResolveToSignalObject=off  FilterRTWStateStorageClass=Auto  ParallelPVariant=InternalParameters  IdealPVariant=Disabled  IVariant=InternalParameters  DVariant=InternalParameters  IntegratorVariant=Discrete  SatVariant=Disabled  AWVariant=Passthrough  PCopyVariant=Disabled  TRVariant=Disabled  FdbkBlocksVariant=Forward  IdealPFdbkVariant=Disabled  SatFdbkVariant=Disabled  DerivativeFilterVariant=ForwardEulerFilter  NVariant=InternalParameters  NCopyVariant=Disabled  FilterICVariant=InternalICsFilter  IntegratorICVariant=InternalICs  ExternalResetVariant=Disabled  TRSumVariant=Passthrough  SumFdbkVariant=Disabled  SumVariant=Sum_PID  TsampFilterVariant=InternalTs  TsampNgainVariant=Passthrough  TsampIntegralVariant=Disabled_SignalSpec  ExternalSaturationOutDataTypeStr=Inherit: Same as second input  DerivativeSourceVariant=ErrorSignal  PreIntVariant=InternalPreInt
  Altitude controller : Subsystem
  Climb Rate SP Merge : Merge
  Climb Rate SP from Guidance : Subsystem  TreatAsAtomicUnit=on
  Compare To Constant : simulink/Logic and Bit Operations/Compare To Constant  relop===  const=uint8(1)  OutDataTypeStr=boolean
  Compare To Constant1 : simulink/Logic and Bit Operations/Compare To Constant  relop===  const=uint8(2)  OutDataTypeStr=boolean
  Pitch SP Controller : Subsystem
  Sum1 : Sum  Inputs=|+-
  Pitch SP : Outport
  Throttle : Outport  Port=2
  wires:
  Airspeed SP/1 -> Sum1/1
  Sum1/1 -> Airspeed Controller/1
  Airspeed/1 -> Sum1/2
  Airspeed Controller/1 -> Throttle/1
  Altitude SP/1 -> Altitude controller/1(Alt SP)
  xyz/1 -> Altitude controller/2(xyz)
  vxyz/1 -> Pitch SP Controller/2(vxyz)
  Pitch SP Controller/1(Pitch SP) -> Pitch SP/1
  Control Mode/1 -> Compare To Constant1/1, Compare To Constant/1
  Compare To Constant/1 -> Altitude controller/Enable
  Compare To Constant1/1 -> Climb Rate SP from Guidance/Enable
  Altitude controller/1(Climb Rate SP) -> Climb Rate SP Merge/1
  Climb Rate SP from Guidance/1(Out1) -> Climb Rate SP Merge/2
  Climb Rate SP Merge/1 -> Pitch SP Controller/1(Climb Rate SP)
  Climb Rate SP/1 -> Climb Rate SP from Guidance/1(Climb Rate SP)

== system UAM_Flight_control/Controller/Auto1/Fixed Wing Controller/Subsystem/Attitude Controller ==
  YPR SP : Inport
  ypr : Inport  Port=2
  Ang Rate : Inport  Port=3
  Airspeed : Inport  Port=4
  Enable : EnablePort  ShowOutputPort=on
  AER Merge : Merge
  Compare To Constant : simulink/Logic and Bit Operations/Compare To Constant  relop===  const=uint8(1)  OutDataTypeStr=boolean
  Compare To Constant1 : simulink/Logic and Bit Operations/Compare To Constant  relop===  const=uint8(2)  OutDataTypeStr=boolean
  Demux1 : Demux  Outputs=3
  Pitch Roll Controller : Subsystem
  Rudder Heading Controller : Subsystem
  AER : Outport
  wires:
  ypr/1 -> Rudder Heading Controller/2(YPR), Pitch Roll Controller/3(YPR)
  YPR SP/1 -> Demux1/1
  Enable/1 -> Compare To Constant1/1, Compare To Constant/1
  AER Merge/1 -> AER/1
  Compare To Constant/1 -> Pitch Roll Controller/Enable
  Pitch Roll Controller/1(AER) -> AER Merge/1
  Rudder Heading Controller/1(AER) -> AER Merge/2
  Demux1/1 -> Rudder Heading Controller/1(Yaw SP)
  Demux1/2 -> Pitch Roll Controller/1(Pitch SP)
  Demux1/3 -> Pitch Roll Controller/2(Roll SP)
  Ang Rate/1 -> Rudder Heading Controller/3(Ang Rate), Pitch Roll Controller/4(Ang Rate)
  Compare To Constant1/1 -> Rudder Heading Controller/Enable
  Airspeed/1 -> Pitch Roll Controller/5(Airspeed)

== system UAM_Flight_control/Controller/Auto1/Fixed Wing Controller/Subsystem/Lateral Guidance Logic ==
  note: S. Park, J. Deyst, and J. P. How, "A New Nonlinear Guidance Logic for Trajectory Tracking," Proceedings of the AIAA Guidance, Navigation and Control Conference, Aug 2004. AIAA-2004-4900.
  Course SP : Inport
  L1 Distance : Inport  Port=2
  course : Inport  Port=3
  gndspeed : Inport  Port=4
  Enable : EnablePort
  Display{,1..3} (4 alike) : Display
  MATLAB Function : MATLAB Function  TreatAsAtomicUnit=on  SystemSampleTime=ControlSampleTime
  Terminator : Terminator
  Roll SP : Outport
  wires:
  course/1 -> Display1/1, MATLAB Function/2(course)
  MATLAB Function/2(rollSP) -> Roll SP/1
  MATLAB Function/1(lacc) -> Terminator/1
  gndspeed/1 -> Display2/1, MATLAB Function/3(groundSpeed)
  L1 Distance/1 -> Display3/1, MATLAB Function/4(L1)
  Course SP/1 -> Display/1, MATLAB Function/1(courseSP)

== system UAM_Flight_control/Controller/Auto1/Fixed Wing Controller/Subsystem/Pitch, Airspeed SP from Controller ==
  Pitch SP In : Inport
  Airspeed SP : Inport  Port=2
  Airspeed : Inport  Port=3
  Enable : EnablePort
  Airspeed Controller : slpidlib/PID Controller  Controller=PID  Form=Parallel  TimeDomain=Discrete-time  UseExternalTs=off  SampleTime=ControlSampleTime  IntegratorMethod=Trapezoidal  FilterMethod=Forward Euler  ControllerParametersSource=internal  P=FWControlParams.P_AIRSPD  I=FWControlParams.I_AIRSPD*0  UseKiTs=off  D=FWControlParams.D_AIRSPD*0  UseExternalDerivativeSource=off  N=FWControlParams.N_AIRSPD  UseFilter=on  TunerSelectOption=Transfer Function Based (PID Tuner App)  InitialConditionSource=internal  InitialConditionForIntegrator=0  InitialConditionForFilter=0  DifferentiatorICPrevScaledInput=0  ExternalReset=none  TrackingMode=off  Kt=1  LimitOutput=off  SatLimitsSource=internal  UpperSaturationLimit=Inf  LowerSaturationLimit=0  LinearizeAsGain=on  AntiWindupMode=clamping  Kb=1  LimitIntegrator=off  UpperIntegratorSaturationLimit=inf  LowerIntegratorSaturationLimit=-inf  POutMin=[]  POutMax=[]  IOutMin=[]  IOutMax=[]  DOutMin=[]  DOutMax=[]  NOutMin=[]  NOutMax=[]  SumOutMin=[]  SumOutMax=[]  SaturationOutMin=[]  SaturationOutMax=[]  PParamMin=[]  PParamMax=[]  IParamMin=[]  IParamMax=[]  DParamMin=[]  DParamMax=[]  NParamMin=[]  NParamMax=[]  KbParamMin=[]  KbParamMax=[]  KtParamMin=[]  KtParamMax=[]  KbOutMin=[]  KbOutMax=[]  KtOutMin=[]  KtOutMax=[]  IntegratorOutMin=[]  IntegratorOutMax=[]  FilterOutMin=[]  FilterOutMax=[]  SumI1OutMin=[]  SumI1OutMax=[]  SumI2OutMin=[]  SumI2OutMax=[]  SumI3OutMin=[]  SumI3OutMax=[]  SumI4OutMin=[]  SumI4OutMax=[]  SumDOutMin=[]  SumDOutMax=[]  DifferentiatorOutMin=[]  DifferentiatorOutMax=[]  FilterDiffOutCoefMin=[]  FilterDiffOutCoefMax=[]  ReciprocalOutMin=[]  ReciprocalOutMax=[]  SumDenOutMin=[]  SumDenOutMax=[]  SumNumOutMin=[]  SumNumOutMax=[]  DivideOutMin=[]  DivideOutMax=[]  UdiffTsProdOutMin=[]  UdiffTsProdOutMax=[]  NTsProdOutMin=[]  NTsProdOutMax=[]  UintegralTsProdOutMin=[]  UintegralTsProdOutMax=[]  UngainTsProdOutMin=[]  UngainTsProdOutMax=[]  ClampingZeroOutDataTypeStr=Inherit: Inherit via back propagation  ClampingZeroOutMin=[]  ClampingZeroOutMax=[]  FilterDenConstantOutDataTypeStr=Inherit: Inherit via back propagation  FilterDenConstantOutMin=[]  FilterDenConstantOutMax=[]  PCopyOutDataTypeStr=Inherit: Inherit via back propagation  PCopyOutMin=[]  PCopyOutMax=[]  NCopyOutDataTypeStr=Inherit: Inherit via back propagation  NCopyOutMin=[]  NCopyOutMax=[]  IntegratorContinuousStateAttributes=''  IntegratorStateMustResolveToSignalObject=off  IntegratorRTWStateStorageClass=Auto  FilterContinuousStateAttributes=''  FilterStateMustResolveToSignalObject=off  FilterRTWStateStorageClass=Auto  ParallelPVariant=InternalParameters  IdealPVariant=Disabled  IVariant=InternalParameters  DVariant=InternalParameters  IntegratorVariant=Discrete  SatVariant=Disabled  AWVariant=Passthrough  PCopyVariant=Disabled  TRVariant=Disabled  FdbkBlocksVariant=Forward  IdealPFdbkVariant=Disabled  SatFdbkVariant=Disabled  DerivativeFilterVariant=ForwardEulerFilter  NVariant=InternalParameters  NCopyVariant=Disabled  FilterICVariant=InternalICsFilter  IntegratorICVariant=InternalICs  ExternalResetVariant=Disabled  TRSumVariant=Passthrough  SumFdbkVariant=Disabled  SumVariant=Sum_PID  TsampFilterVariant=InternalTs  TsampNgainVariant=Passthrough  TsampIntegralVariant=Disabled_SignalSpec  ExternalSaturationOutDataTypeStr=Inherit: Same as second input  DerivativeSourceVariant=ErrorSignal  PreIntVariant=InternalPreInt
  IC : InitialCondition  Value=0
  Sum1 : Sum  Inputs=|+-
  Pitch SP : Outport
  Throttle : Outport  Port=2
  wires:
  IC/1 -> Pitch SP/1
  Pitch SP In/1 -> IC/1
  Airspeed SP/1 -> Sum1/1
  Sum1/1 -> Airspeed Controller/1
  Airspeed/1 -> Sum1/2
  Airspeed Controller/1 -> Throttle/1

== system UAM_Flight_control/Controller/Auto1/Fixed Wing Controller/Subsystem/Roll SP from Path Manager ==
  In1 : Inport
  Enable : EnablePort
  IC : InitialCondition  Value=0
  Out1 : Outport
  wires:
  In1/1 -> IC/1
  IC/1 -> Out1/1

== system UAM_Flight_control/Controller/Auto1/Fixed Wing Controller/Subsystem/Subsystem2 ==
  Euler : Inport
  pqr : Inport  Port=2
  Demux : Demux  Outputs=3
  MATLAB Function : MATLAB Function  TreatAsAtomicUnit=on
  Terminator : Terminator
  Terminator1 : Terminator
  Euler Rate : Outport
  wires:
  Demux/1 -> MATLAB Function/1(phi)
  Demux/2 -> MATLAB Function/2(theta)
  MATLAB Function/1(y) -> Terminator1/1
  pqr/1 -> Euler Rate/1
  Euler/1 -> Demux/1
  Demux/3 -> Terminator/1

== system UAM_Flight_control/Controller/Auto1/Multicopter Controller/Attitude & Altitude controller/Altitude Control ==
  note: commanded thrust = PD(e_vz)
  note: e_vz = Vz_ref +(– Vz)
  note: Vz_ref = Kp_z * e_z
  note: e_z = Z_cmd - Z_out
  note: in1 : false일때 출력
      | in2 : 조건
      | in3: true일떄 출력
  note: InTrasition 상태일때 동작
  note: Maintain altitude previously set when in transition
  States : Inport
  Z ref : Inport  Port=2
  InTransition : Inport  Port=3
  FlightMode : Inport  Port=4
  Enable : EnablePort  StatesWhenEnabling=reset  ShowOutputPort=on
  Altitude controller : slpidlib/PID Controller  Controller=P  Form=Parallel  TimeDomain=Discrete-time  UseExternalTs=off  SampleTime=-1  IntegratorMethod=Forward Euler  FilterMethod=Forward Euler  ControllerParametersSource=internal  P=controlParams.P_Z  I=controlParams.I_Z  UseKiTs=off  D=controlParams.D_Z  UseExternalDerivativeSource=off  N=controlParams.N_Z  UseFilter=on  TunerSelectOption=Transfer Function Based (PID Tuner App)  InitialConditionSource=internal  InitialConditionForIntegrator=0  InitialConditionForFilter=0  DifferentiatorICPrevScaledInput=0  ExternalReset=none  TrackingMode=off  Kt=1  LimitOutput=on  SatLimitsSource=internal  UpperSaturationLimit=5  LowerSaturationLimit=-5  LinearizeAsGain=on  AntiWindupMode=none  Kb=1  LimitIntegrator=off  UpperIntegratorSaturationLimit=inf  LowerIntegratorSaturationLimit=-inf  POutMin=[]  POutMax=[]  IOutMin=[]  IOutMax=[]  DOutMin=[]  DOutMax=[]  NOutMin=[]  NOutMax=[]  SumOutMin=[]  SumOutMax=[]  SaturationOutMin=[]  SaturationOutMax=[]  PParamMin=[]  PParamMax=[]  IParamMin=[]  IParamMax=[]  DParamMin=[]  DParamMax=[]  NParamMin=[]  NParamMax=[]  KbParamMin=[]  KbParamMax=[]  KtParamMin=[]  KtParamMax=[]  KbOutMin=[]  KbOutMax=[]  KtOutMin=[]  KtOutMax=[]  IntegratorOutMin=[]  IntegratorOutMax=[]  FilterOutMin=[]  FilterOutMax=[]  SumI1OutMin=[]  SumI1OutMax=[]  SumI2OutMin=[]  SumI2OutMax=[]  SumI3OutMin=[]  SumI3OutMax=[]  SumI4OutMin=[]  SumI4OutMax=[]  SumDOutMin=[]  SumDOutMax=[]  DifferentiatorOutMin=[]  DifferentiatorOutMax=[]  FilterDiffOutCoefMin=[]  FilterDiffOutCoefMax=[]  ReciprocalOutMin=[]  ReciprocalOutMax=[]  SumDenOutMin=[]  SumDenOutMax=[]  SumNumOutMin=[]  SumNumOutMax=[]  DivideOutMin=[]  DivideOutMax=[]  UdiffTsProdOutMin=[]  UdiffTsProdOutMax=[]  NTsProdOutMin=[]  NTsProdOutMax=[]  UintegralTsProdOutMin=[]  UintegralTsProdOutMax=[]  UngainTsProdOutMin=[]  UngainTsProdOutMax=[]  ClampingZeroOutDataTypeStr=Inherit: Inherit via back propagation  ClampingZeroOutMin=[]  ClampingZeroOutMax=[]  FilterDenConstantOutDataTypeStr=Inherit: Inherit via back propagation  FilterDenConstantOutMin=[]  FilterDenConstantOutMax=[]  PCopyOutDataTypeStr=Inherit: Inherit via back propagation  PCopyOutMin=[]  PCopyOutMax=[]  NCopyOutDataTypeStr=Inherit: Inherit via back propagation  NCopyOutMin=[]  NCopyOutMax=[]  IntegratorContinuousStateAttributes=''  IntegratorStateMustResolveToSignalObject=off  IntegratorRTWStateStorageClass=Auto  FilterContinuousStateAttributes=''  FilterStateMustResolveToSignalObject=off  FilterRTWStateStorageClass=Auto  ParallelPVariant=InternalParameters  IdealPVariant=Disabled  IVariant=Disabled  DVariant=Disabled  IntegratorVariant=Disabled  SatVariant=Enabled  AWVariant=Disabled  PCopyVariant=Disabled  TRVariant=Disabled  FdbkBlocksVariant=Forward  IdealPFdbkVariant=Disabled  SatFdbkVariant=Disabled  DerivativeFilterVariant=Disabled  NVariant=Disabled  NCopyVariant=Disabled_SignalSpec  FilterICVariant=Disabled  IntegratorICVariant=Disabled  ExternalResetVariant=Disabled  TRSumVariant=Passthrough  SumFdbkVariant=Disabled  SumVariant=Passthrough_P  TsampFilterVariant=InternalTs  TsampNgainVariant=Passthrough  TsampIntegralVariant=Disabled_SignalSpec  ExternalSaturationOutDataTypeStr=Inherit: Same as second input  DerivativeSourceVariant=Disabled  PreIntVariant=InternalPreInt
  Altitude rate controller1 : slpidlib/PID Controller  Controller=PID  Form=Parallel  TimeDomain=Discrete-time  UseExternalTs=off  SampleTime=-1  IntegratorMethod=Forward Euler  FilterMethod=Forward Euler  ControllerParametersSource=internal  P=controlParams.P_VZ  I=controlParams.I_VZ  UseKiTs=off  D=controlParams.D_VZ  UseExternalDerivativeSource=off  N=controlParams.N_VZ  UseFilter=on  TunerSelectOption=Transfer Function Based (PID Tuner App)  InitialConditionSource=internal  InitialConditionForIntegrator=0  InitialConditionForFilter=0  DifferentiatorICPrevScaledInput=0  ExternalReset=rising  TrackingMode=off  Kt=1  LimitOutput=on  SatLimitsSource=internal  UpperSaturationLimit=inf  LowerSaturationLimit=-inf  LinearizeAsGain=on  AntiWindupMode=clamping  Kb=1  LimitIntegrator=on  UpperIntegratorSaturationLimit=2  LowerIntegratorSaturationLimit=-1.5  POutMin=[]  POutMax=[]  IOutMin=[]  IOutMax=[]  DOutMin=[]  DOutMax=[]  NOutMin=[]  NOutMax=[]  SumOutMin=[]  SumOutMax=[]  SaturationOutMin=[]  SaturationOutMax=[]  PParamMin=[]  PParamMax=[]  IParamMin=[]  IParamMax=[]  DParamMin=[]  DParamMax=[]  NParamMin=[]  NParamMax=[]  KbParamMin=[]  KbParamMax=[]  KtParamMin=[]  KtParamMax=[]  KbOutMin=[]  KbOutMax=[]  KtOutMin=[]  KtOutMax=[]  IntegratorOutMin=[]  IntegratorOutMax=[]  FilterOutMin=[]  FilterOutMax=[]  SumI1OutMin=[]  SumI1OutMax=[]  SumI2OutMin=[]  SumI2OutMax=[]  SumI3OutMin=[]  SumI3OutMax=[]  SumI4OutMin=[]  SumI4OutMax=[]  SumDOutMin=[]  SumDOutMax=[]  DifferentiatorOutMin=[]  DifferentiatorOutMax=[]  FilterDiffOutCoefMin=[]  FilterDiffOutCoefMax=[]  ReciprocalOutMin=[]  ReciprocalOutMax=[]  SumDenOutMin=[]  SumDenOutMax=[]  SumNumOutMin=[]  SumNumOutMax=[]  DivideOutMin=[]  DivideOutMax=[]  UdiffTsProdOutMin=[]  UdiffTsProdOutMax=[]  NTsProdOutMin=[]  NTsProdOutMax=[]  UintegralTsProdOutMin=[]  UintegralTsProdOutMax=[]  UngainTsProdOutMin=[]  UngainTsProdOutMax=[]  ClampingZeroOutDataTypeStr=Inherit: Inherit via back propagation  ClampingZeroOutMin=[]  ClampingZeroOutMax=[]  FilterDenConstantOutDataTypeStr=Inherit: Inherit via back propagation  FilterDenConstantOutMin=[]  FilterDenConstantOutMax=[]  PCopyOutDataTypeStr=Inherit: Inherit via back propagation  PCopyOutMin=[]  PCopyOutMax=[]  NCopyOutDataTypeStr=Inherit: Inherit via back propagation  NCopyOutMin=[]  NCopyOutMax=[]  IntegratorContinuousStateAttributes=''  IntegratorStateMustResolveToSignalObject=off  IntegratorRTWStateStorageClass=Auto  FilterContinuousStateAttributes=''  FilterStateMustResolveToSignalObject=off  FilterRTWStateStorageClass=Auto  ParallelPVariant=InternalParameters  IdealPVariant=Disabled  IVariant=InternalParameters  DVariant=InternalParameters  IntegratorVariant=Discrete  SatVariant=Enabled  AWVariant=DiscClampingParallel  PCopyVariant=Disabled  TRVariant=Disabled  FdbkBlocksVariant=Forward  IdealPFdbkVariant=Disabled  SatFdbkVariant=Disabled  DerivativeFilterVariant=ForwardEulerFilter  NVariant=InternalParameters  NCopyVariant=Disabled  FilterICVariant=InternalICsFilter  IntegratorICVariant=InternalICs  ExternalResetVariant=ExternalReset  TRSumVariant=Passthrough  SumFdbkVariant=Disabled  SumVariant=Sum_PID  TsampFilterVariant=InternalTs  TsampNgainVariant=Passthrough  TsampIntegralVariant=Disabled_SignalSpec  ExternalSaturationOutDataTypeStr=Inherit: Same as second input  DerivativeSourceVariant=ErrorSignal  PreIntVariant=InternalPreInt
  Bus Selector : BusSelector  OutputSignals=Xe,Ve,Abb
  Constant4 : Constant  Value=flightState.FixedWing
  Cos : Trigonometry  Operator=cos
  Cos1 : Trigonometry  Operator=cos
  Demux : Demux  Outputs=3
  Display8 : Display
  Display9 : Display
  Divide : Product  Inputs=*/
  Equal : RelationalOperator  Operator===  OutDataTypeStr=boolean  RndMeth=Simplest  InputSameDT=off
  Gain : Gain  Gain=-1
  Gain1 : Gain  Gain=-1
  MATLAB Function : MATLAB Function  TreatAsAtomicUnit=on
  NOT : Logic  Operator=NOT  IconShape=distinctive  AllPortsSameDT=off  OutDataTypeStr=boolean
  Product : Product
  Product1 : Product
  Saturation1 : Saturate  UpperLimit=0.9  LowerLimit=0.15
  Selector : Selector  InputPortWidth=3  IndexOptions=Index vector (dialog)  Indices=[3]  OutputSizes=1
  Selector1 : Selector  InputPortWidth=3  IndexOptions=Index vector (dialog)  Indices=[3]  OutputSizes=1
  Sum : Sum  Inputs=|+-
  Sum1 : Sum  Inputs=|+-
  Sum3 : Sum  Inputs=|++
  Switch : Switch  Criteria=u2 > Threshold  SaturateOnIntegerOverflow=off  InputSameDT=off
  Switch1 : Switch  Criteria=u2 > Threshold  SaturateOnIntegerOverflow=off  InputSameDT=off
  Triggered Subsystem : Subsystem  TreatAsAtomicUnit=on
  Unary Minus : UnaryMinus
  Unit Delay : UnitDelay  SampleTime=-1  HasFrameUpgradeWarning=on
  hover_thrust/g : Gain  Gain=1/9.81
  commanded thrust : Outport
  wires:
  States/1 -> Bus Selector/1
  InTransition/1 -> NOT/1, Triggered Subsystem/Trigger
  Switch/1 -> Unary Minus/1  "Output"
  NOT/1 -> Switch/2
  Triggered Subsystem/1(Reference) -> Switch1/1, Switch/3  "Stable"
  Bus Selector/1 -> Selector/1  "<Xe>"
  Bus Selector/2 -> Selector1/1  "<Ve>"
  Altitude controller/1 -> Sum1/1
  Constant4/1 -> Equal/1
  FlightMode/1 -> Equal/2
  Equal/1 -> Switch1/2
  Z ref/1 -> Switch1/3
  Switch1/1 -> Switch/1  "Output"
  Sum/1 -> Altitude controller/1
  Selector1/1 -> Gain1/1
  Selector/1 -> Gain/1, Triggered Subsystem/1(AltHold)
  Gain/1 -> Sum/2
  Gain1/1 -> [vz], Sum1/2
  Enable/1 -> [active]
  [active] -> Altitude rate controller1/2
  Altitude rate controller1/1 -> Product1/2  "thrust"
  [phi] -> Cos/1
  MATLAB Function/1(hover_est) -> Product1/1, Sum3/2
  [active] -> MATLAB Function/4(active)
  [vz] -> MATLAB Function/2(vz)
  Product/1 -> Divide/2, Display8/1
  [az] -> MATLAB Function/3(az)
  hover_thrust/g/1 -> Sum3/1
  Sum3/1 -> Divide/1, Display9/1
  Product1/1 -> hover_thrust/g/1
  Cos1/1 -> Product/2
  Divide/1 -> Saturation1/1
  Sum1/1 -> Altitude rate controller1/1
  Saturation1/1 -> commanded thrust/1, Unit Delay/1
  Cos/1 -> Product/1
  Unit Delay/1 -> MATLAB Function/1(thrust_in)
  [theta] -> Cos1/1
  Bus Selector/3 -> Demux/1  "<Abb>"
  Demux/3 -> [az]
  Unary Minus/1 -> Sum/1
